simulink model "MLIB_Sub_BAM_F32"  (Simulink 8.3)
settings: Solver=ode45  StartTime=0.0  StopTime=10.0  RelTol=1e-3
settings Model: Creator=RE004C  LastModifiedBy=B17364
settings OptimizationCC: ExpressionDepthLimit=2147483647
settings DebuggingCC: FcnCallInpInsideContextMsg=UseLocalSettings  StrictBusMsg=Warning
settings HardwareCC: ProdLargestAtomicInteger=Long  ProdLargestAtomicFloat=Double  ProdIntDivRoundTo=Zero  ProdEndianess=BigEndian  ProdHWDeviceType=Freescale->32-bit PowerPC

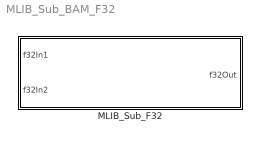
== system MLIB_Sub_BAM_F32 ==
  MLIB_Sub_F32 : Subsystem  mask(MLIB_Sub_F32){}
      mask help: Bit accurate model of subtract of two input values. All parameters as well as input and output are 32bit integers.
      mask init:
      | pos = get_param(gcb, 'Position');width = pos(3) - pos(1); height = pos(4) - pos(2);tX=width/2;tY=height*0.9;
      mask Display: color('black');port_label('input',1,'f32In1');port_label('input',2,'f32In2');port_label('output',1,'f32Out');color('black');disp('MLIB_Sub_F32');color('blue');text(tX,tY, 'BAM', 'horizontalAlignment', 'center');

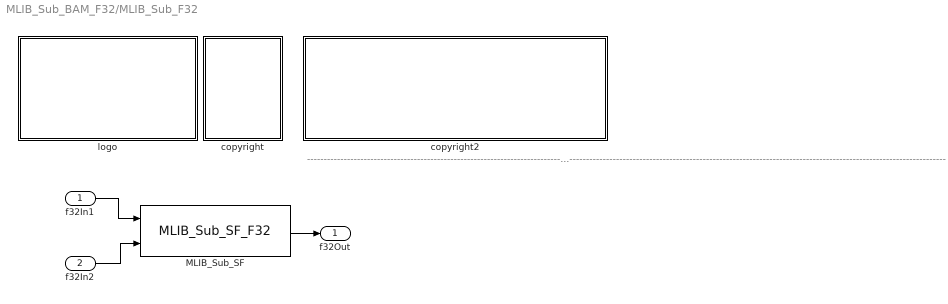
== system MLIB_Sub_BAM_F32/MLIB_Sub_F32 ==
  note: ---------------------------------------------------------------------------------------------------------------------------------------------------------------------------------------------------
  f32In1 : Inport
  f32In2 : Inport  Port=2
  MLIB_Sub_SF : S-Function  FunctionName=MLIB_Sub_SF_F32  EnableBusSupport=off
  copyright : Subsystem
      mask Display:
      | text(10,90,'FILE:');text(10,75,'DESRIPTION:')
      | text(10,60,'COPYRIGHT:')
      | text(10,45,'VERSION:')
      | text(10,30,'DATE:')
  copyright2 : Subsystem
      mask Display:
      | text(10,90,'MLIB_Sub_BAM_F32.mdl');text(10,75,'Sum of two input values.');text(10,60,'Freescale')
      | text(10,45,'0.1');text(10,30,'18-Jul-2011');
  logo : Subsystem
      mask Display: image(imread('logo.jpg'))
  f32Out : Outport
  wires:
  f32In1/1 -> MLIB_Sub_SF/1
  f32In2/1 -> MLIB_Sub_SF/2
  MLIB_Sub_SF/1 -> f32Out/1

== system MLIB_Sub_BAM_F32/MLIB_Sub_F32/copyright ==

== system MLIB_Sub_BAM_F32/MLIB_Sub_F32/copyright2 ==

== system MLIB_Sub_BAM_F32/MLIB_Sub_F32/logo ==
